simulink model "SIRVE"  (Simulink 9.0)
settings: Solver=VariableStepAuto  StartTime=0.0  StopTime=10.0  RelTol=1e-3
libraries: instrumentlib x2
settings Model: Creator=oscar  LastModifiedBy=oscar
settings DataIOCC: SaveFormat=Dataset
settings OptimizationCC: LifeSpan=auto
settings DebuggingCC: UnderspecifiedInitializationDetection=Simplified  MergeDetectMultiDrivingBlocksExec=error  SFUnexpectedBacktrackingDiag=error  SFNoUnconditionalDefaultTransitionDiag=error  SFExecutionAtInitializationDiag=warning
settings HardwareCC: ProdBitPerPointer=64  ProdBitPerSizeT=64  ProdBitPerPtrDiffT=64  ProdLargestAtomicFloat=Float  ProdIntDivRoundTo=Zero  ProdEndianess=LittleEndian  ProdWordSize=64  ProdHWDeviceType=Intel->x86-64 (Windows64)
settings ModelReferenceCC: PropagateSignalLabelsOutOfModel=on
settings CodeAppCC: StateflowObjectComments=off
settings GRTTargetCC: TargetLangStandard=C99 (ISO)
settings ConfigComp: CovMetricSettings=dwe  CovHtmlReporting=off  CovSaveCumulativeToWorkspaceVar=off  CovSaveSingleToWorkspaceVar=off  CovExternalEMLEnable=on

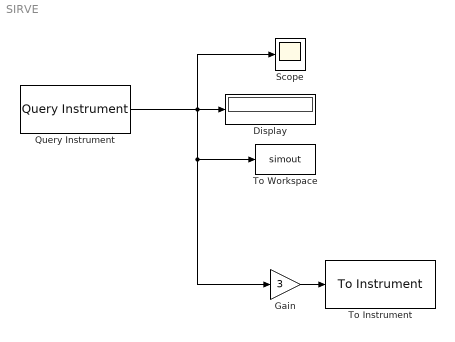
== system SIRVE ==
  Display : Display
  Gain : Gain  Gain=3
  Query Instrument : instrumentlib/Query Instrument  sampleTime=0.5  isWorkspaceObject=off  timeout=10  inputBufferSize=512  protocol=Serial  serialPort=COM3  baudRate=9600  gpibVendor=Agilent Technologies  boardIndex=0  primaryAddress=1  secondaryAddress=0  visaVendor=Agilent  visaSerialPort=0  chassisIndex=0  logicalAddress=0  tcpRemoteHost='127.0.0.1'  tcpRemotePort=4500  udpRemoteHost='127.0.0.1'  udpRemotePort=9090  visaTCPBoardIndex=0  visaTCPRemoteHost='127.0.0.1'  usbBoardIndex=0  usbManufID=0  usbModelCode=0  usbSerialNumber=0  initAction=None  initCommand='DATA:SOURCE CH1'  initFunction=get  queryCommand=''  responseFormat=ASCII  asciiFormatting='%d,'  precision=8-bit integer  byteOrder=Little endian  valuesToRead=1  removeBytes=off  afterOutputAction=Repeat query for new data  enableFrames=on  frameSize=1
      settings: SourceProductName=Instrument Control Toolbox  SourceProductBaseCode=IC
  Scope : Scope
  To Instrument : instrumentlib/To Instrument  sampleTime=-1  isWorkspaceObject=off  timeout=10  inputBufferSize=8192  protocol=Serial  serialPort=COM3  baudRate=9600  gpibVendor=Agilent Technologies  boardIndex=0  primaryAddress=1  secondaryAddress=0  visaVendor=Agilent  visaSerialPort=0  chassisIndex=0  logicalAddress=0  tcpRemoteHost='127.0.0.1'  tcpRemotePort=4500  udpRemoteHost='127.0.0.1'  udpRemotePort=9090  visaTCPBoardIndex=0  visaTCPRemoteHost='127.0.0.1'  usbBoardIndex=0  usbManufID=0  usbModelCode=0  usbSerialNumber=0  initAction=None  initCommand='DATA:SOURCE CH1'  initFunction=get  command=''  sendFormat=Binary  asciiFormatting='%d'  precision=8-bit integer  byteOrder=Little endian
      settings: SourceProductName=Instrument Control Toolbox  SourceProductBaseCode=IC
  To Workspace : ToWorkspace  VariableName=simout  SaveFormat=Timeseries  SampleTime=-1
  wires:
  Query Instrument/1 -> Gain/1, To Workspace/1, Scope/1, Display/1
  Gain/1 -> To Instrument/1
